simulink model "ArchitectureControleNavigation"  (R2023b)
settings: Solver=ode8  StartTime=0.0  StopTime=Duree  FixedStep=0.1  RelTol=1e-3  EnableMultiTasking=on
values from neighbouring files (symbols this model uses):
  AccelerationAngulaireMax = 1    [matlab.mat]
  AccelerationLineaireMax = 1    [matlab.mat]
settings Model: Creator=Lounis Adouane  LastModifiedBy=User
settings SolverCC: AlgebraicLoopSolver=TrustRegion
settings DataIOCC: LimitDataPoints=on  SaveFormat=Array  SignalLoggingSaveFormat=ModelDataLogs  ReturnWorkspaceOutputs=off  SignalLoggingName=sigsOut
settings OptimizationCC: InitFltsAndDblsToZero=on  LifeSpan=inf
settings DebuggingCC: AlgebraicLoopMsg=none  SaveWithParameterizedLinksMsg=none  UnderspecifiedInitializationDetection=Classic  MergeDetectMultiDrivingBlocksExec=none  SignalResolutionControl=TryResolveAllWithWarning  MultiTaskDSMMsg=warning  MultiTaskCondExecSysMsg=none  UnconnectedInputMsg=warning  UnconnectedOutputMsg=warning  UnconnectedLineMsg=warning  SFUnexpectedBacktrackingDiag=warning  SFNoUnconditionalDefaultTransitionDiag=warning  SFExecutionAtInitializationDiag=none  ArithmeticOperatorsInVariantConditions=warning
settings HardwareCC: ProdBitPerPointer=32  ProdBitPerSizeT=32  ProdBitPerPtrDiffT=32  ProdLargestAtomicFloat=None  ProdIntDivRoundTo=Undefined  ProdEndianess=Unspecified  ProdWordSize=32  ProdHWDeviceType=32-bit Generic  TargetUnknown=on
settings ModelReferenceCC: PropagateSignalLabelsOutOfModel=off
settings SFSimCC: SimUseLocalCustomCode=off  CustomCodeUndefinedFunction=UseInterfaceOnly
settings RTWCC: RTWUseLocalCustomCode=off
settings CodeAppCC: StateflowObjectComments=on
settings GRTTargetCC: TargetFcnLib=ansi_tfl_tmw.mat  TargetLangStandard=C89/C90 (ANSI)  CombineOutputUpdateFcns=off  GRTInterface=on
settings ConfigComp: CovMetricSettings=dw  CovSaveCumulativeToWorkspaceVar=on  CovSaveSingleToWorkspaceVar=on  CovExternalEMLEnable=off

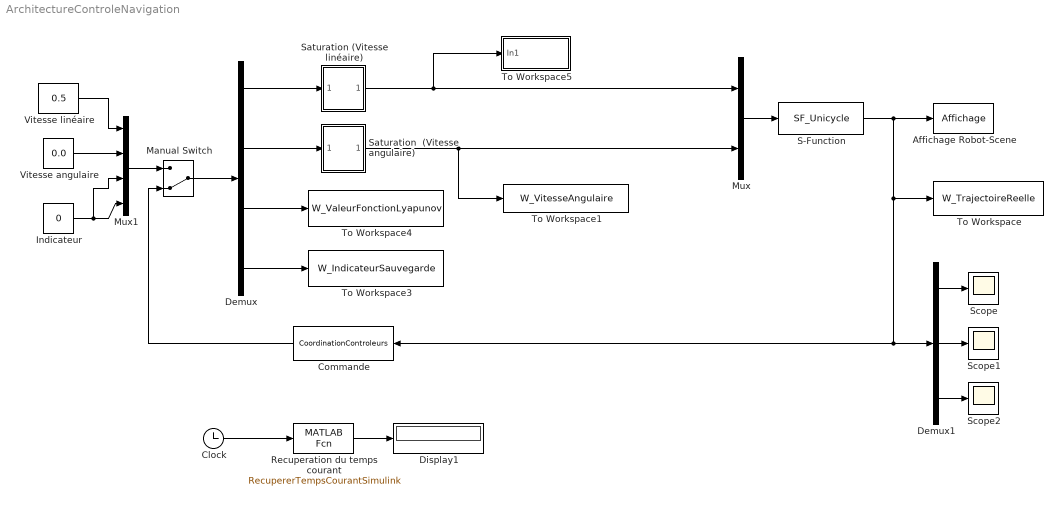
== system ArchitectureControleNavigation ==
  Affichage Robot-Scene : MATLABFcn  MATLABFcn=Affichage  OutputDimensions=0
  Clock : Clock
  "Commande " : MATLABFcn  MATLABFcn=CoordinationControleurs
  Demux : Demux
  Demux1 : Demux  Outputs=3
  Display1 : Display
  Indicateur : Constant  Value=0
  Manual Switch : ManualSwitch  CurrentSetting=0
  Mux : Mux  Inputs=2
  Mux1 : Mux
  Recuperation du temps courant : MATLABFcn  MATLABFcn=RecupererTempsCourantSimulink  OutputSignalType=real
  S-Function : S-Function  FunctionName=SF_Unicycle  Parameters=Xreel0, Yreel0, Theta0  SFunctionDeploymentMode=off  EnableBusSupport=off
  "Saturation  (Vitesse angulaire) " : Subsystem
  Saturation (Vitesse linéaire) : Subsystem
  Scope : Scope
  Scope1 : Scope
  Scope2 : Scope
  To Workspace : ToWorkspace  VariableName=W_TrajectoireReelle  SampleTime=-1
  To Workspace1 : ToWorkspace  VariableName=W_VitesseAngulaire  SampleTime=-1
  To Workspace3 : ToWorkspace  VariableName=W_IndicateurSauvegarde  SampleTime=-1
  To Workspace4 : ToWorkspace  VariableName=W_ValeurFonctionLyapunov  SampleTime=-1
  To Workspace5 : Subsystem
  Vitesse angulaire : Constant  Value=0.0
  Vitesse linéaire : Constant  Value=0.5
  wires:
  S-Function/1 -> "Commande "/1, Demux1/1, To Workspace/1, Affichage Robot-Scene/1
  Mux/1 -> S-Function/1
  Clock/1 -> Recuperation du temps courant/1
  Recuperation du temps courant/1 -> Display1/1
  Saturation (Vitesse linéaire)/1(Out1) -> To Workspace5/1(In1), Mux/1
  Demux/2 -> "Saturation  (Vitesse angulaire) "/1(In1)
  Demux/1 -> Saturation (Vitesse linéaire)/1(In1)
  Vitesse linéaire/1 -> Mux1/1
  Vitesse angulaire/1 -> Mux1/2
  Mux1/1 -> Manual Switch/1
  "Commande "/1 -> Manual Switch/2
  Manual Switch/1 -> Demux/1
  Demux1/1 -> Scope/1
  Demux1/2 -> Scope1/1
  Demux1/3 -> Scope2/1
  "Saturation  (Vitesse angulaire) "/1(Out1) -> To Workspace1/1, Mux/2
  Indicateur/1 -> Mux1/4, Mux1/3
  Demux/4 -> To Workspace3/1
  Demux/3 -> To Workspace4/1

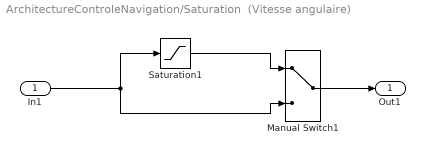
== system ArchitectureControleNavigation/Saturation  (Vitesse angulaire)  ==
  In1 : Inport
  Manual Switch1 : ManualSwitch
  Saturation1 : Saturate  UpperLimit=AccelerationAngulaireMax  LowerLimit=-AccelerationAngulaireMax
  Out1 : Outport
  wires:
  In1/1 -> Manual Switch1/2, Saturation1/1
  Saturation1/1 -> Manual Switch1/1
  Manual Switch1/1 -> Out1/1

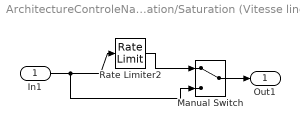
== system ArchitectureControleNavigation/Saturation (Vitesse linéaire) ==
  In1 : Inport
  Manual Switch : ManualSwitch
  Rate Limiter2 : RateLimiter  RisingSlewLimit=AccelerationLineaireMax  FallingSlewLimit=-AccelerationLineaireMax  SampleTimeMode=inherited
  Out1 : Outport
  wires:
  In1/1 -> Manual Switch/2, Rate Limiter2/1
  Rate Limiter2/1 -> Manual Switch/1
  Manual Switch/1 -> Out1/1

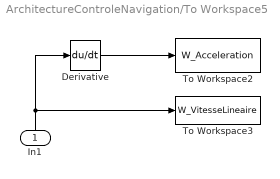
== system ArchitectureControleNavigation/To Workspace5 ==
  In1 : Inport
  Derivative : Derivative
  To Workspace2 : ToWorkspace  VariableName=W_Acceleration  SampleTime=-1
  To Workspace3 : ToWorkspace  VariableName=W_VitesseLineaire  SampleTime=-1
  wires:
  Derivative/1 -> To Workspace2/1
  In1/1 -> Derivative/1, To Workspace3/1
